simulink model "satelit_mdl"  (R2024a)
settings: Solver=VariableStepAuto  StartTime=0.0  StopTime=1800  RelTol=1e-3
values from neighbouring files (symbols this model uses):
  dr1_0 = [4953.572247 -3787.24327881 -4362.50090206]    [constants.mat]
  dr2_0 = [5448.9294717 -4165.96760669 -4798.75099227]    [constants.mat]
  epsilon0 = 1e4    (= 10000)    [Satelit.m]
  r1_0 = [-3111566.74666 2420733.54744 -5626803.09256]    [constants.mat]
  r2_0 = alpha + r2_0_copy    [Satelit.m]    (also in constants.mat = [-3422723.42133 2662806.90219 -6189483.40182])
settings Model: Creator=User  LastModifiedBy=User

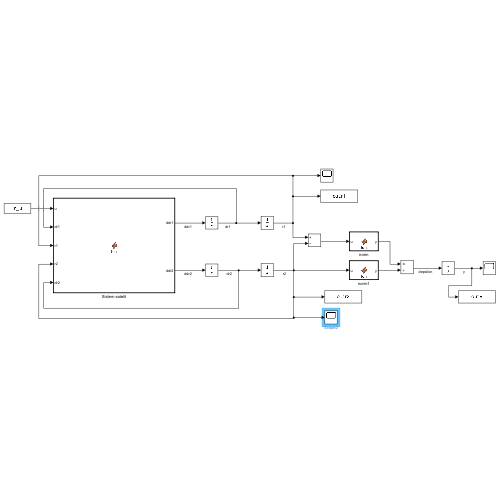
[thumbnail: Simulink's stored preview of the top-level diagram]
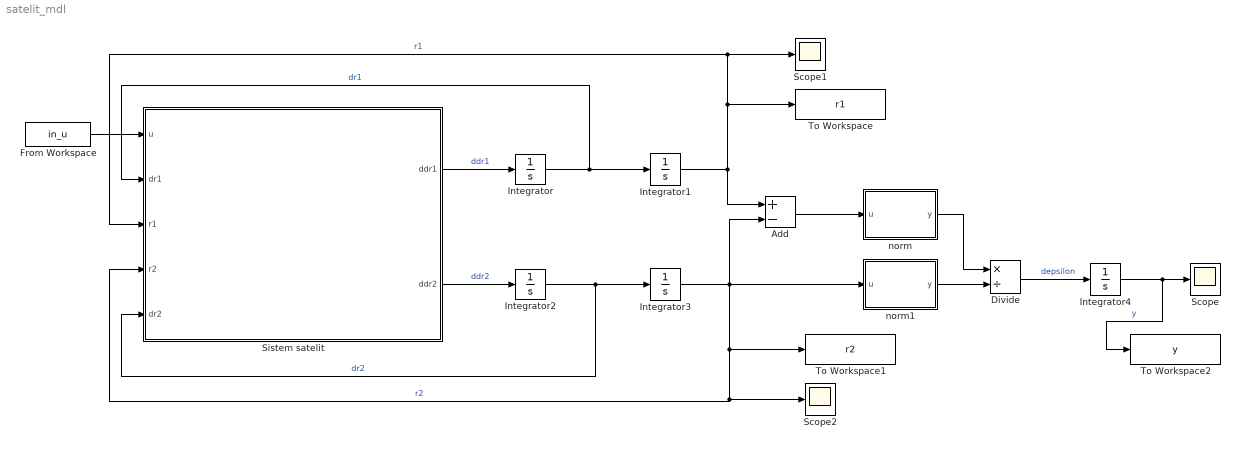
== system satelit_mdl ==
  Add : Sum  Inputs=+-
  Divide : Product  Inputs=*/  RndMeth=Zero  SaturateOnIntegerOverflow=on
  From Workspace : FromWorkspace  VariableName=in_u
  Integrator : Integrator  InitialCondition=dr1_0
  Integrator1 : Integrator  InitialCondition=r1_0
  Integrator2 : Integrator  InitialCondition=dr2_0
  Integrator3 : Integrator  InitialCondition=r2_0
  Integrator4 : Integrator  InitialCondition=epsilon0
  Scope : Scope
  Scope1 : Scope
  Scope2 : Scope
  Sistem satelit : MATLAB Function  TreatAsAtomicUnit=on
  To Workspace : ToWorkspace  VariableName=r1  SaveFormat=Timeseries  SampleTime=-1
  To Workspace1 : ToWorkspace  VariableName=r2  SaveFormat=Timeseries  SampleTime=-1
  To Workspace2 : ToWorkspace  VariableName=y  SaveFormat=Timeseries  SampleTime=-1
  norm : MATLAB Function  TreatAsAtomicUnit=on
  norm1 : MATLAB Function  TreatAsAtomicUnit=on
  wires:
  Sistem satelit/1(ddr1) -> Integrator/1  "ddr1"
  Sistem satelit/2(ddr2) -> Integrator2/1  "ddr2"
  Integrator/1 -> Sistem satelit/2(dr1), Integrator1/1  "dr1"
  Integrator2/1 -> Integrator3/1, Sistem satelit/5(dr2)  "dr2"
  Integrator1/1 -> Sistem satelit/3(r1), Scope1/1, To Workspace/1, Add/1  "r1"
  Integrator3/1 -> Add/2, norm1/1(u), Scope2/1, Sistem satelit/4(r2), To Workspace1/1  "r2"
  Add/1 -> norm/1(u)
  norm/1(y) -> Divide/1
  norm1/1(y) -> Divide/2
  Divide/1 -> Integrator4/1  "depsilon"
  Integrator4/1 -> To Workspace2/1, Scope/1  "y"
  From Workspace/1 -> Sistem satelit/1(u)

== matlab function satelit_mdl/norm ==
  data: u input; y output
function y = fcn(u)

y = norm(u);

== matlab function satelit_mdl/Sistem satelit ==
  data: u input; dr1 input; r1 input; ddr1 output; r2 input; dr2 input; ddr2 output
function [ddr1, ddr2]= fcn(u, dr1, r1, r2, dr2)

G = 6.674e-11;
Mp = 5.972e24;
Rp = 6371000;
J2 = 1.08262668e-3;
omegap = 7.2921e-5;

ddr1 = -((G*Mp)/norm(r1)^2) .* (r1/norm(r1)) - ...
       (3/2 * J2 * G * Mp * Rp^2 / norm(r1)^5) .* ...
       [(r1(1) - 5 * r1(1) * r1(3)^2)/norm(r1)^2;
        (r1(2) - 5 * r1(2) * r1(3)^2)/norm(r1)^2;
        (r1(3) - 5 * r1(3) * r1(3)^2)/norm(r1)^2] + ...
        omegap^2 .* [r1(1); r1(2); 0] + ...
        2*omegap .* [dr1(2); -dr1(1); 0] + ...
        u;

ddr2 = -((G*Mp)/norm(r2)^2) .* (r2/norm(r2)) - ...
       (3/2 * J2 * G * Mp * Rp^2 / norm(r2)^5) .* ...
       [(r2(1) - 5 * r2(1) * r2(3)^2)/norm(r2)^2;
        (r2(2) - 5 * r2(2) * r2(3)^2)/norm(r2)^2;
        (r2(3) - 5 * r2(3) * r2(3)^2)/norm(r2)^2] + ...
        omegap^2 .* [r2(1); r2(2); 0] + ...
        2*omegap .* [dr2(2); -dr2(1); 0];

== matlab function satelit_mdl/norm1 ==
  data: u input; y output
function y = fcn(u)

y = norm(u);
